simulink model "CSuntitled"  (Simulink 6.0)
settings: Solver=ode45  StartTime=0.0  StopTime=7  RelTol=1e-3
settings Model: LastModifiedBy=John

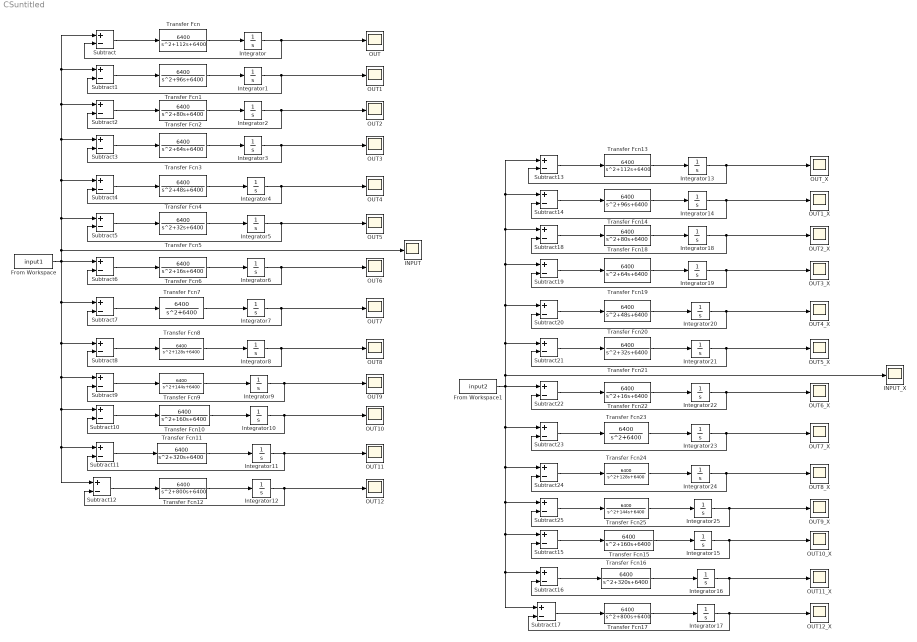
== system CSuntitled ==
  From Workspace : FromWorkspace  VariableName=input1  SampleTime=0
  From Workspace1 : FromWorkspace  VariableName=input2  SampleTime=0
  INPUT : Scope
      settings: SaveName=INPUT  DataFormat=Array
  INPUT_X : Scope
      settings: SaveName=INPUT_X  DataFormat=Array
  Integrator{,1..12} (13 alike) : Integrator
  Integrator{13..25} (13 alike) : Integrator  InitialCondition=1
  OUT{,1..12} (13 alike) : Scope
      OUT settings: SaveName=OUT  DataFormat=Array
      OUT1 settings: SaveName=OUT1  DataFormat=Array
      OUT10 settings: SaveName=OUT10  DataFormat=Array
      OUT11 settings: SaveName=OUT11  DataFormat=Array
      OUT12 settings: SaveName=OUT12  DataFormat=Array
      OUT2 settings: SaveName=OUT2  DataFormat=Array
      OUT3 settings: SaveName=OUT3  DataFormat=Array
      OUT4 settings: SaveName=OUT4  DataFormat=Array
      OUT5 settings: SaveName=OUT5  DataFormat=Array
      OUT6 settings: SaveName=OUT6  DataFormat=Array
      OUT7 settings: SaveName=OUT7  DataFormat=Array
      OUT8 settings: SaveName=OUT8  DataFormat=Array
      OUT9 settings: SaveName=OUT9  DataFormat=Array
  OUT10_X : Scope
      settings: SaveName=OUT10_X  DataFormat=Array
  OUT11_X : Scope
      settings: SaveName=OUT11_X  DataFormat=Array
  OUT12_X : Scope
      settings: SaveName=OUT12_X  DataFormat=Array
  OUT1_X : Scope
      settings: SaveName=OUT1_X  DataFormat=Array
  OUT2_X : Scope
      settings: SaveName=OUT2_X  DataFormat=Array
  OUT3_X : Scope
      settings: SaveName=OUT3_X  DataFormat=Array
  OUT4_X : Scope
      settings: SaveName=OUT4_X  DataFormat=Array
  OUT5_X : Scope
      settings: SaveName=OUT5_X  DataFormat=Array
  OUT6_X : Scope
      settings: SaveName=OUT6_X  DataFormat=Array
  OUT7_X : Scope
      settings: SaveName=OUT7_X  DataFormat=Array
  OUT8_X : Scope
      settings: SaveName=OUT8_X  DataFormat=Array
  OUT9_X : Scope
      settings: SaveName=OUT9_X  DataFormat=Array
  OUT_X : Scope
      settings: SaveName=OUT_X  DataFormat=Array
  Subtract{,1..25} (26 alike) : Sum  Inputs=+-  OutScaling=2^-10
  Transfer Fcn : TransferFcn  Numerator=[6400]  Denominator=[1 112 6400]
  Transfer Fcn1 : TransferFcn  Numerator=[6400]  Denominator=[1 96 6400]
  Transfer Fcn10 : TransferFcn  Numerator=[6400]  Denominator=[1 160 6400]
  Transfer Fcn11 : TransferFcn  Numerator=[6400]  Denominator=[1 320 6400]
  Transfer Fcn12 : TransferFcn  Numerator=[6400]  Denominator=[1 800 6400]
  Transfer Fcn13 : TransferFcn  Numerator=[6400]  Denominator=[1 112 6400]
  Transfer Fcn14 : TransferFcn  Numerator=[6400]  Denominator=[1 96 6400]
  Transfer Fcn15 : TransferFcn  Numerator=[6400]  Denominator=[1 160 6400]
  Transfer Fcn16 : TransferFcn  Numerator=[6400]  Denominator=[1 320 6400]
  Transfer Fcn17 : TransferFcn  Numerator=[6400]  Denominator=[1 800 6400]
  Transfer Fcn18 : TransferFcn  Numerator=[6400]  Denominator=[1 80 6400]
  Transfer Fcn19 : TransferFcn  Numerator=[6400]  Denominator=[1 64 6400]
  Transfer Fcn2 : TransferFcn  Numerator=[6400]  Denominator=[1 80 6400]
  Transfer Fcn20 : TransferFcn  Numerator=[6400]  Denominator=[1 48 6400]
  Transfer Fcn21 : TransferFcn  Numerator=[6400]  Denominator=[1 32 6400]
  Transfer Fcn22 : TransferFcn  Numerator=[6400]  Denominator=[1 16 6400]
  Transfer Fcn23 : TransferFcn  Numerator=[6400]  Denominator=[1 0 6400]
  Transfer Fcn24 : TransferFcn  Numerator=[6400]  Denominator=[1 128 6400]
  Transfer Fcn25 : TransferFcn  Numerator=[6400]  Denominator=[1 144 6400]
  Transfer Fcn3 : TransferFcn  Numerator=[6400]  Denominator=[1 64 6400]
  Transfer Fcn4 : TransferFcn  Numerator=[6400]  Denominator=[1 48 6400]
  Transfer Fcn5 : TransferFcn  Numerator=[6400]  Denominator=[1 32 6400]
  Transfer Fcn6 : TransferFcn  Numerator=[6400]  Denominator=[1 16 6400]
  Transfer Fcn7 : TransferFcn  Numerator=[6400]  Denominator=[1 0 6400]
  Transfer Fcn8 : TransferFcn  Numerator=[6400]  Denominator=[1 128 6400]
  Transfer Fcn9 : TransferFcn  Numerator=[6400]  Denominator=[1 144 6400]
  wires:
  Subtract/1 -> Transfer Fcn/1
  Transfer Fcn/1 -> Integrator/1
  From Workspace/1 -> Subtract6/1, Subtract7/1, Subtract8/1, Subtract9/1, Subtract10/1, Subtract12/1, Subtract11/1, Subtract/1, Subtract1/1, Subtract2/1, Subtract3/1, Subtract4/1, Subtract5/1, INPUT/1
  Integrator/1 -> Subtract/2, OUT/1
  Integrator1/1 -> Subtract1/2, OUT1/1
  Transfer Fcn1/1 -> Integrator1/1
  Subtract1/1 -> Transfer Fcn1/1
  Subtract2/1 -> Transfer Fcn2/1
  Transfer Fcn2/1 -> Integrator2/1
  Subtract3/1 -> Transfer Fcn3/1
  Transfer Fcn3/1 -> Integrator3/1
  Integrator2/1 -> Subtract2/2, OUT2/1
  Integrator3/1 -> Subtract3/2, OUT3/1
  Subtract4/1 -> Transfer Fcn4/1
  Transfer Fcn4/1 -> Integrator4/1
  Integrator4/1 -> Subtract4/2, OUT4/1
  Subtract5/1 -> Transfer Fcn5/1
  Transfer Fcn5/1 -> Integrator5/1
  Integrator5/1 -> Subtract5/2, OUT5/1
  Subtract6/1 -> Transfer Fcn6/1
  Transfer Fcn6/1 -> Integrator6/1
  Integrator6/1 -> Subtract6/2, OUT6/1
  Subtract7/1 -> Transfer Fcn7/1
  Transfer Fcn7/1 -> Integrator7/1
  Integrator7/1 -> Subtract7/2, OUT7/1
  Subtract8/1 -> Transfer Fcn8/1
  Transfer Fcn8/1 -> Integrator8/1
  Subtract9/1 -> Transfer Fcn9/1
  Transfer Fcn9/1 -> Integrator9/1
  Integrator8/1 -> Subtract8/2, OUT8/1
  Subtract10/1 -> Transfer Fcn10/1
  Integrator9/1 -> Subtract9/2, OUT9/1
  Transfer Fcn10/1 -> Integrator10/1
  Integrator10/1 -> Subtract10/2, OUT10/1
  Subtract11/1 -> Transfer Fcn11/1
  Transfer Fcn11/1 -> Integrator11/1
  Integrator11/1 -> Subtract11/2, OUT11/1
  Subtract12/1 -> Transfer Fcn12/1
  Transfer Fcn12/1 -> Integrator12/1
  Integrator12/1 -> Subtract12/2, OUT12/1
  Subtract13/1 -> Transfer Fcn13/1
  Transfer Fcn13/1 -> Integrator13/1
  From Workspace1/1 -> Subtract22/1, Subtract23/1, Subtract24/1, Subtract25/1, Subtract15/1, Subtract17/1, Subtract16/1, Subtract13/1, Subtract14/1, Subtract18/1, Subtract19/1, Subtract20/1, Subtract21/1, INPUT_X/1
  Integrator13/1 -> Subtract13/2, OUT_X/1
  Integrator14/1 -> Subtract14/2, OUT1_X/1
  Transfer Fcn14/1 -> Integrator14/1
  Subtract14/1 -> Transfer Fcn14/1
  Subtract18/1 -> Transfer Fcn18/1
  Transfer Fcn18/1 -> Integrator18/1
  Subtract19/1 -> Transfer Fcn19/1
  Transfer Fcn19/1 -> Integrator19/1
  Integrator18/1 -> Subtract18/2, OUT2_X/1
  Integrator19/1 -> Subtract19/2, OUT3_X/1
  Subtract20/1 -> Transfer Fcn20/1
  Transfer Fcn20/1 -> Integrator20/1
  Integrator20/1 -> Subtract20/2, OUT4_X/1
  Subtract21/1 -> Transfer Fcn21/1
  Transfer Fcn21/1 -> Integrator21/1
  Integrator21/1 -> Subtract21/2, OUT5_X/1
  Subtract22/1 -> Transfer Fcn22/1
  Transfer Fcn22/1 -> Integrator22/1
  Integrator22/1 -> Subtract22/2, OUT6_X/1
  Subtract23/1 -> Transfer Fcn23/1
  Transfer Fcn23/1 -> Integrator23/1
  Integrator23/1 -> Subtract23/2, OUT7_X/1
  Subtract24/1 -> Transfer Fcn24/1
  Transfer Fcn24/1 -> Integrator24/1
  Subtract25/1 -> Transfer Fcn25/1
  Transfer Fcn25/1 -> Integrator25/1
  Integrator24/1 -> Subtract24/2, OUT8_X/1
  Subtract15/1 -> Transfer Fcn15/1
  Integrator25/1 -> Subtract25/2, OUT9_X/1
  Transfer Fcn15/1 -> Integrator15/1
  Integrator15/1 -> Subtract15/2, OUT10_X/1
  Subtract16/1 -> Transfer Fcn16/1
  Transfer Fcn16/1 -> Integrator16/1
  Integrator16/1 -> Subtract16/2, OUT11_X/1
  Subtract17/1 -> Transfer Fcn17/1
  Transfer Fcn17/1 -> Integrator17/1
  Integrator17/1 -> Subtract17/2, OUT12_X/1
